simulink model "ex14_eval"  (R2023a)
settings: Solver=ode45  StartTime=0.0  StopTime=tfinal  MaxStep=1e-3  RelTol=1e-3  EnableMultiTasking=on
values from neighbouring files (symbols this model uses):
  h = 'Digital Filter $\tilde{G}_{1}$(s)'    [ex13.m]    (also in ex14.m = 0.2)
  K2 = dlqr(A2,B2,Q2,R2,N2)    [ex14.m]
  pca = [2,-1;1,0]    [ex14.m]
  pcb = [1;0]    [ex14.m]
  pcc = [0,1]    [ex14.m]
  pcd = 0    [ex14.m]
  x0 = [1; -2; 2; -1]    [ex05.m]    (also in ex11.m = inv(z*eye(3)-A)*B*u0; ex11_2.m = inv(z*eye(3)-A)*B*u0; ex14.m = [10;1])
settings Model: Creator=瀬部昇  LastModifiedBy=vigro
settings SolverCC: AlgebraicLoopSolver=TrustRegion
settings DataIOCC: LimitDataPoints=on  SaveFormat=Array  SignalLoggingSaveFormat=ModelDataLogs  ReturnWorkspaceOutputs=off
settings OptimizationCC: ExpressionDepthLimit=2147483647  InitFltsAndDblsToZero=on  LifeSpan=inf
settings DebuggingCC: UnderspecifiedInitializationDetection=Classic  MergeDetectMultiDrivingBlocksExec=none  SolverPrmCheckMsg=warning  FcnCallInpInsideContextMsg=warning  UnconnectedInputMsg=warning  UnconnectedOutputMsg=warning  UnconnectedLineMsg=warning  StateNameClashWarn=warning  SFUnexpectedBacktrackingDiag=warning  SFNoUnconditionalDefaultTransitionDiag=warning  SFExecutionAtInitializationDiag=none  ArithmeticOperatorsInVariantConditions=warning
settings HardwareCC: ProdBitPerPointer=32  ProdBitPerSizeT=32  ProdBitPerPtrDiffT=32  ProdLargestAtomicFloat=None  ProdIntDivRoundTo=Undefined  ProdEndianess=Unspecified  ProdWordSize=32  ProdHWDeviceType=32-bit Generic
settings ModelReferenceCC: EnableRefExpFcnMdlSchedulingChecks=on  PropagateSignalLabelsOutOfModel=off
settings RTWCC: DLArmComputeVersion=19.05
settings CodeAppCC: StateflowObjectComments=on
settings GRTTargetCC: TargetLangStandard=C89/C90 (ANSI)  CombineOutputUpdateFcns=off  GRTInterface=on
settings ConfigComp: CovMetricSettings=dw  CovSaveCumulativeToWorkspaceVar=on  CovSaveSingleToWorkspaceVar=on

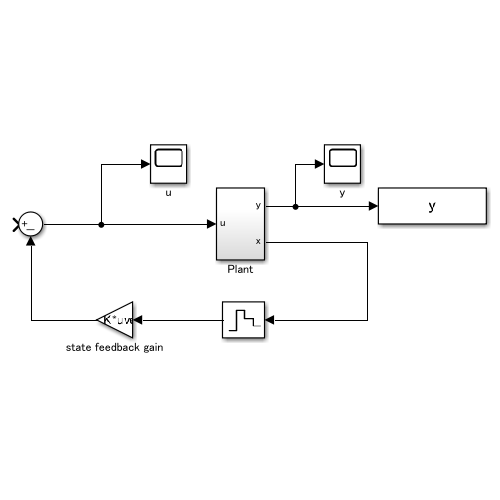
[thumbnail: Simulink's stored preview of the top-level diagram]
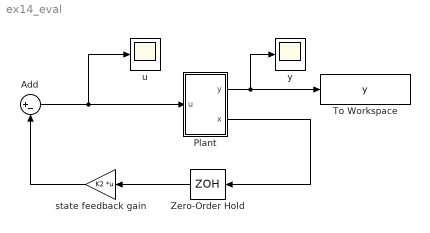
== system ex14_eval ==
  Add : Sum  Inputs=|+-
  Plant : Subsystem
  To Workspace : ToWorkspace  VariableName=y  SaveFormat=Structure With Time  SampleTime=1e-2
  Zero-Order Hold : ZeroOrderHold  SampleTime=h
  state feedback gain : Gain  Gain=K2  Multiplication=Matrix(K*u) (u vector)
  u : Scope
  y : Scope
  wires:
  Plant/2(x) -> Zero-Order Hold/1
  Plant/1(y) -> y/1, To Workspace/1
  Zero-Order Hold/1 -> state feedback gain/1
  state feedback gain/1 -> Add/2
  Add/1 -> u/1, Plant/1(u)

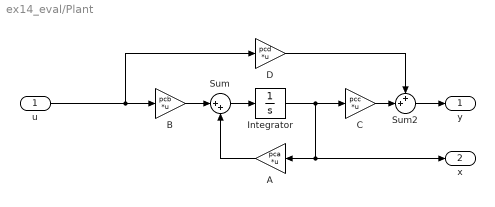
== system ex14_eval/Plant ==
  u : Inport
  A : Gain  Gain=pca  Multiplication=Matrix(K*u) (u vector)
  B : Gain  Gain=pcb  Multiplication=Matrix(K*u) (u vector)
  C : Gain  Gain=pcc  Multiplication=Matrix(K*u) (u vector)
  D : Gain  Gain=pcd  Multiplication=Matrix(K*u) (u vector)
  Integrator : Integrator  InitialCondition=x0
  Sum : Sum  Inputs=|++
  Sum2 : Sum  Inputs=++|
  y : Outport
  x : Outport  Port=2
  wires:
  Sum/1 -> Integrator/1
  Integrator/1 -> C/1, A/1, x/1
  A/1 -> Sum/2
  B/1 -> Sum/1
  u/1 -> B/1, D/1
  D/1 -> Sum2/1
  C/1 -> Sum2/2
  Sum2/1 -> y/1
